simulink model "M4B11"  (R2016b)
settings: Solver=VariableStepAuto  StartTime=0.0  StopTime=25  RelTol=1e-3
InitFcn:
  | initAll
values from neighbouring files (symbols this model uses):
  SgridB = resultsac.baseMVA    [initAll.m]
  wB = 2*pi*fB    (= 314.159265359)    [initAll.m]
undefined symbols (not defined in the file): ACgirdinit, Geninit
libraries: powerlib_meascontrol x4
(part 1 of 2)
settings Model: Creator=LinSiQi  LastModifiedBy=LinSiQi
settings DataIOCC: ReturnWorkspaceOutputs=on
settings SFSimCC: SimUseLocalCustomCode=on
settings RTWCC: RTWUseLocalCustomCode=on

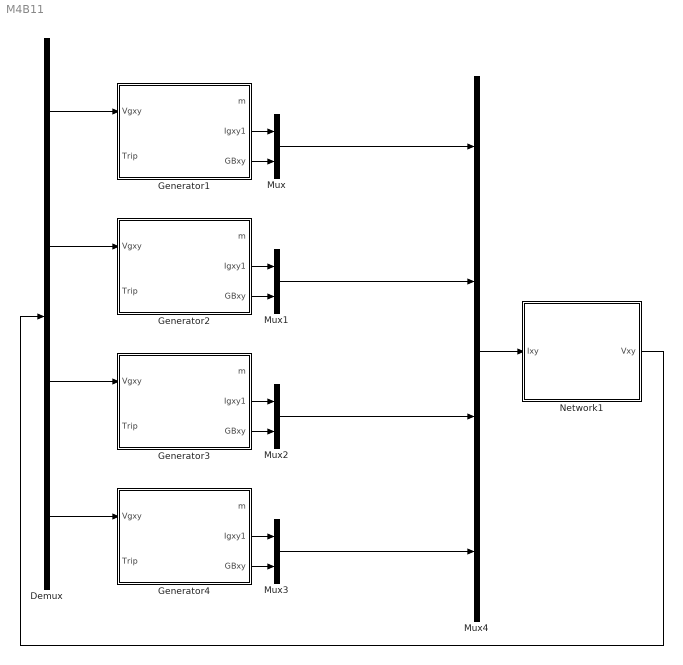
== system M4B11 ==
  Demux : Demux
  Generator1 : Subsystem  mask{wB=wB, SgenB=Geninit.SgenB(1), SgridB=SgridB, Xq=Geninit.Xq(1), Xq1=Geninit.Xq1(1), Xq11=Geninit.Xq11(1), Tq0=Geninit.Tq0(1), Tq10=Geninit.Tq10(1), Eq10=Geninit.Eq1(1), Eq110=Geninit.Eq11(1), Xd=Geninit.Xd(1), Xd1=Geninit.Xd1(1), Xd11=Geninit.Xd11(1), Td0=Geninit.Td0(1), Td10=Geninit.Td10(1), Ed10=Geninit.Ed1(1), Ed110=Geninit.Ed11(1), H=Geninit.Tj(1), D=Geninit.D(1), delta0=Geninit.Delta(1), w0=1, Pm0=Geninit.Pm0(1), Ka=Geninit.Ka(1), Tb=Geninit.Tb(1), Tc=Geninit.Tc(1), Efmin=Geninit.Efmin(1), Efmax=Geninit.Efmax(1), Vref=Geninit.Vref(1), Ef10=Geninit.Vf1(1), S_PSS=Geninit.EnablePSS(1), Kpss=Geninit.kpss(1), Tw_P=Geninit.Tw_P(1), T1_P=Geninit.T1_P(1), T2_P=Geninit.T2_P(1), T3_P=Geninit.T3_P(1), T4_P=Geninit.T4_P(1), Upmax=Geninit.Upmax(1), Upmin=Geninit.Upmin(1), S_Gov=Geninit.Enablegov(1), R=Geninit.R_G(1), Ts_G=Geninit.Ts_G(1), Tc_G=Geninit.Tc_G(1), T3_G=Geninit.T3_G(1), T4_G=Geninit.T4_G(1), T5_G=Geninit.T5_G(1), dPmax=Geninit.dPmax(1), dPmin=Geninit.dPmin(1)}
      mask prompts: S_PSS "Enable PSS"; Tw_P "Tw"; T1_P "T1"; T2_P "T2"; T3_P "T3"; T4_P "T4"; S_Gov "Enable Governor"; Ts_G "Ts"; Tc_G "Tc"; T3_G "T3"; T4_G "T4"; T5_G "T5"
      mask help: This is a six-order synchronous generator with exciter system, governor and PSS.
  Generator2 : Subsystem  mask{wB=wB, SgenB=Geninit.SgenB(2), SgridB=SgridB, Xq=Geninit.Xq(2), Xq1=Geninit.Xq1(2), Xq11=Geninit.Xq11(2), Tq0=Geninit.Tq0(2), Tq10=Geninit.Tq10(2), Eq10=Geninit.Eq1(2), Eq110=Geninit.Eq11(2), Xd=Geninit.Xd(2), Xd1=Geninit.Xd1(2), Xd11=Geninit.Xd11(2), Td0=Geninit.Td0(2), Td10=Geninit.Td10(2), Ed10=Geninit.Ed1(2), Ed110=Geninit.Ed11(2), H=Geninit.Tj(2), D=Geninit.D(2), delta0=Geninit.Delta(2), w0=1, Pm0=Geninit.Pm0(2), Ka=Geninit.Ka(2), Tb=Geninit.Tb(2), Tc=Geninit.Tc(2), Efmin=Geninit.Efmin(2), Efmax=Geninit.Efmax(2), Vref=Geninit.Vref(2), Ef10=Geninit.Vf1(2), S_PSS=Geninit.EnablePSS(2), Kpss=Geninit.kpss(2), Tw_P=Geninit.Tw_P(2), T1_P=Geninit.T1_P(2), T2_P=Geninit.T2_P(2), T3_P=Geninit.T3_P(2), T4_P=Geninit.T4_P(2), Upmax=Geninit.Upmax(2), Upmin=Geninit.Upmin(2), S_Gov=Geninit.Enablegov(2), R=Geninit.R_G(2), Ts_G=Geninit.Ts_G(2), Tc_G=Geninit.Tc_G(2), T3_G=Geninit.T3_G(2), T4_G=Geninit.T4_G(2), T5_G=Geninit.T5_G(2), dPmax=Geninit.dPmax(2), dPmin=Geninit.dPmin(2)}
      mask prompts: S_PSS "Enable PSS"; Tw_P "Tw"; T1_P "T1"; T2_P "T2"; T3_P "T3"; T4_P "T4"; S_Gov "Enable Governor"; Ts_G "Ts"; Tc_G "Tc"; T3_G "T3"; T4_G "T4"; T5_G "T5"
      mask help: This is a six-order synchronous generator with exciter system, governor and PSS.
  Generator3 : Subsystem  mask{wB=wB, SgenB=Geninit.SgenB(3), SgridB=SgridB, Xq=Geninit.Xq(3), Xq1=Geninit.Xq1(3), Xq11=Geninit.Xq11(3), Tq0=Geninit.Tq0(3), Tq10=Geninit.Tq10(3), Eq10=Geninit.Eq1(3), Eq110=Geninit.Eq11(3), Xd=Geninit.Xd(3), Xd1=Geninit.Xd1(3), Xd11=Geninit.Xd11(3), Td0=Geninit.Td0(3), Td10=Geninit.Td10(3), Ed10=Geninit.Ed1(3), Ed110=Geninit.Ed11(3), H=Geninit.Tj(3), D=Geninit.D(3), delta0=Geninit.Delta(3), w0=1, Pm0=Geninit.Pm0(3), Ka=Geninit.Ka(3), Tb=Geninit.Tb(3), Tc=Geninit.Tc(3), Efmin=Geninit.Efmin(3), Efmax=Geninit.Efmax(3), Vref=Geninit.Vref(3), Ef10=Geninit.Vf1(3), S_PSS=Geninit.EnablePSS(3), Kpss=Geninit.kpss(3), Tw_P=Geninit.Tw_P(3), T1_P=Geninit.T1_P(3), T2_P=Geninit.T2_P(3), T3_P=Geninit.T3_P(3), T4_P=Geninit.T4_P(3), Upmax=Geninit.Upmax(3), Upmin=Geninit.Upmin(3), S_Gov=Geninit.Enablegov(3), R=Geninit.R_G(3), Ts_G=Geninit.Ts_G(3), Tc_G=Geninit.Tc_G(3), T3_G=Geninit.T3_G(3), T4_G=Geninit.T4_G(3), T5_G=Geninit.T5_G(3), dPmax=Geninit.dPmax(3), dPmin=Geninit.dPmin(3)}
      mask prompts: S_PSS "Enable PSS"; Tw_P "Tw"; T1_P "T1"; T2_P "T2"; T3_P "T3"; T4_P "T4"; S_Gov "Enable Governor"; Ts_G "Ts"; Tc_G "Tc"; T3_G "T3"; T4_G "T4"; T5_G "T5"
      mask help: This is a six-order synchronous generator with exciter system, governor and PSS.
  Generator4 : Subsystem  mask{wB=wB, SgenB=Geninit.SgenB(4), SgridB=SgridB, Xq=Geninit.Xq(4), Xq1=Geninit.Xq1(4), Xq11=Geninit.Xq11(4), Tq0=Geninit.Tq0(4), Tq10=Geninit.Tq10(4), Eq10=Geninit.Eq1(4), Eq110=Geninit.Eq11(4), Xd=Geninit.Xd(4), Xd1=Geninit.Xd1(4), Xd11=Geninit.Xd11(4), Td0=Geninit.Td0(4), Td10=Geninit.Td10(4), Ed10=Geninit.Ed1(4), Ed110=Geninit.Ed11(4), H=Geninit.Tj(4), D=Geninit.D(4), delta0=Geninit.Delta(4), w0=1, Pm0=Geninit.Pm0(4), Ka=Geninit.Ka(4), Tb=Geninit.Tb(4), Tc=Geninit.Tc(4), Efmin=Geninit.Efmin(4), Efmax=Geninit.Efmax(4), Vref=Geninit.Vref(4), Ef10=Geninit.Vf1(4), S_PSS=Geninit.EnablePSS(4), Kpss=Geninit.kpss(4), Tw_P=Geninit.Tw_P(4), T1_P=Geninit.T1_P(4), T2_P=Geninit.T2_P(4), T3_P=Geninit.T3_P(4), T4_P=Geninit.T4_P(4), Upmax=Geninit.Upmax(4), Upmin=Geninit.Upmin(4), S_Gov=Geninit.Enablegov(4), R=Geninit.R_G(4), Ts_G=Geninit.Ts_G(4), Tc_G=Geninit.Tc_G(4), T3_G=Geninit.T3_G(4), T4_G=Geninit.T4_G(4), T5_G=Geninit.T5_G(4), dPmax=Geninit.dPmax(4), dPmin=Geninit.dPmin(4)}
      mask prompts: S_PSS "Enable PSS"; Tw_P "Tw"; T1_P "T1"; T2_P "T2"; T3_P "T3"; T4_P "T4"; S_Gov "Enable Governor"; Ts_G "Ts"; Tc_G "Tc"; T3_G "T3"; T4_G "T4"; T5_G "T5"
      mask help: This is a six-order synchronous generator with exciter system, governor and PSS.
  Mux{,1..3} (4 alike) : Mux  Inputs=2
  Mux4 : Mux
  Network1 : Subsystem  mask{busdata=ACgirdinit.busdata{1}, linedata=ACgirdinit.linedata{1}, VSS0=ACgirdinit.VSS0{1}, LINE=ACgirdinit.fline{1}, fbus=ACgirdinit.FBUS(1), ng=ACgirdinit.ng{1}, Currentin_idx=ACgirdinit.Currentin_idx{1}}
  wires:
  Mux/1 -> Mux4/1
  Generator2/2(Igxy1) -> Mux1/1
  Generator3/2(Igxy1) -> Mux2/1
  Generator1/2(Igxy1) -> Mux/1
  Generator2/3(GBxy) -> Mux1/2
  Mux1/1 -> Mux4/2
  Mux2/1 -> Mux4/3
  Mux3/1 -> Mux4/4
  Generator4/3(GBxy) -> Mux3/2
  Generator4/2(Igxy1) -> Mux3/1
  Generator1/3(GBxy) -> Mux/2
  Generator3/3(GBxy) -> Mux2/2
  Mux4/1 -> Network1/1(Ixy)
  Demux/1 -> Generator1/1(Vgxy)
  Demux/2 -> Generator2/1(Vgxy)
  Demux/3 -> Generator3/1(Vgxy)
  Demux/4 -> Generator4/1(Vgxy)
  Network1/1(Vxy) -> Demux/1

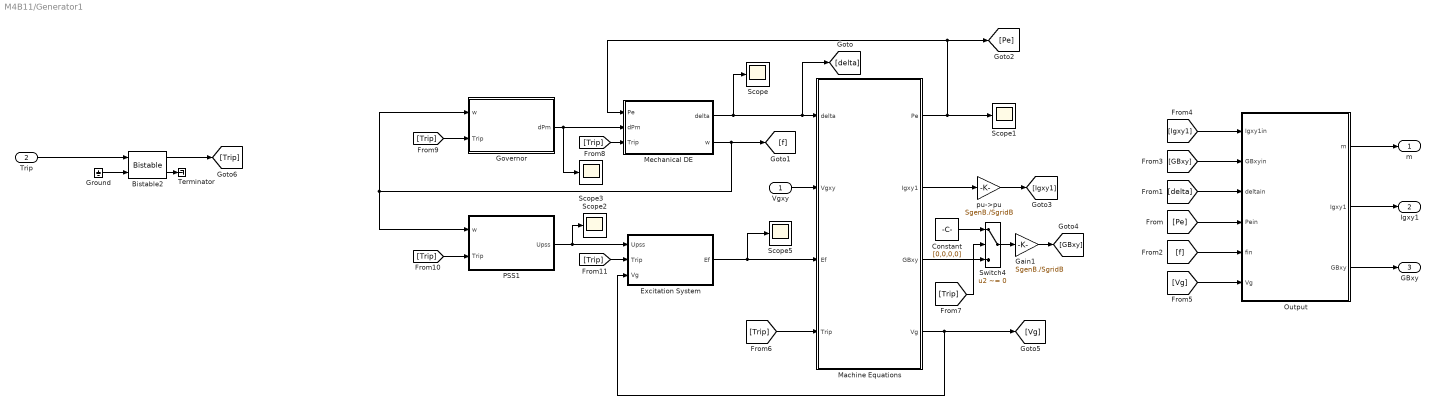
== system M4B11/Generator1 ==
  Vgxy : Inport
  Trip : Inport  Port=2
  Bistable2 : powerlib_meascontrol/Logic/Bistable  Qpriority=Set  ic=0  Ts=0
  Constant : Constant  Value=[0,0,0,0]
  Excitation System : Subsystem
  Gain1 : Gain  Gain=SgenB./SgridB
  Governor : Subsystem
  Ground : Ground
  "Machine Equations " : Subsystem
  Mechanical DE : Subsystem
  Output : Subsystem
  PSS1 : Subsystem
  Scope{,1..3,5} (5 alike) : Scope
  Switch4 : Switch  Criteria=u2 ~= 0  Threshold=0.5  SaturateOnIntegerOverflow=on
  Terminator : Terminator
  pu->pu : Gain  Gain=SgenB./SgridB
  m : Outport
  Igxy1 : Outport  Port=2
  GBxy : Outport  Port=3
  wires:
  Gain1/1 -> [GBxy]
  pu->pu/1 -> [Igxy1]
  [Trip] -> PSS1/2(Trip)
  [Trip] -> Governor/2(Trip)
  [GBxy] -> Output/2(GBxyin)
  [Trip] -> Excitation System/2(Trip)
  Output/1(m) -> m/1
  Mechanical DE/1(delta) -> Scope/1, "Machine Equations "/1(delta), [delta]
  Bistable2/2 -> Terminator/1
  [f] -> Output/5(fin)
  Output/2(Igxy1) -> Igxy1/1
  PSS1/1(Upss) -> Excitation System/1(Upss), Scope2/1
  "Machine Equations "/3(GBxy) -> Switch4/3
  Vgxy/1 -> "Machine Equations "/2(Vgxy)
  Constant/1 -> Switch4/1
  "Machine Equations "/2(Igxy1) -> pu->pu/1
  Governor/1(dPm) -> Mechanical DE/2(dPm), Scope3/1
  [delta] -> Output/3(deltain)
  [Vg] -> Output/6(Vg)
  [Igxy1] -> Output/1(Igxy1in)
  Mechanical DE/2(w) -> Governor/1(w), PSS1/1(w), [f]
  Output/3(GBxy) -> GBxy/1
  Excitation System/1(Ef) -> Scope5/1, "Machine Equations "/3(Ef)
  "Machine Equations "/4(Vg) -> [Vg], Excitation System/3(Vg)
  [Trip] -> "Machine Equations "/4(Trip)
  [Trip] -> Switch4/2
  Bistable2/1 -> [Trip]
  "Machine Equations "/1(Pe) -> Scope1/1, Mechanical DE/1(Pe), [Pe]
  [Pe] -> Output/4(Pein)
  Switch4/1 -> Gain1/1
  Trip/1 -> Bistable2/1
  Ground/1 -> Bistable2/2
  [Trip] -> Mechanical DE/3(Trip)

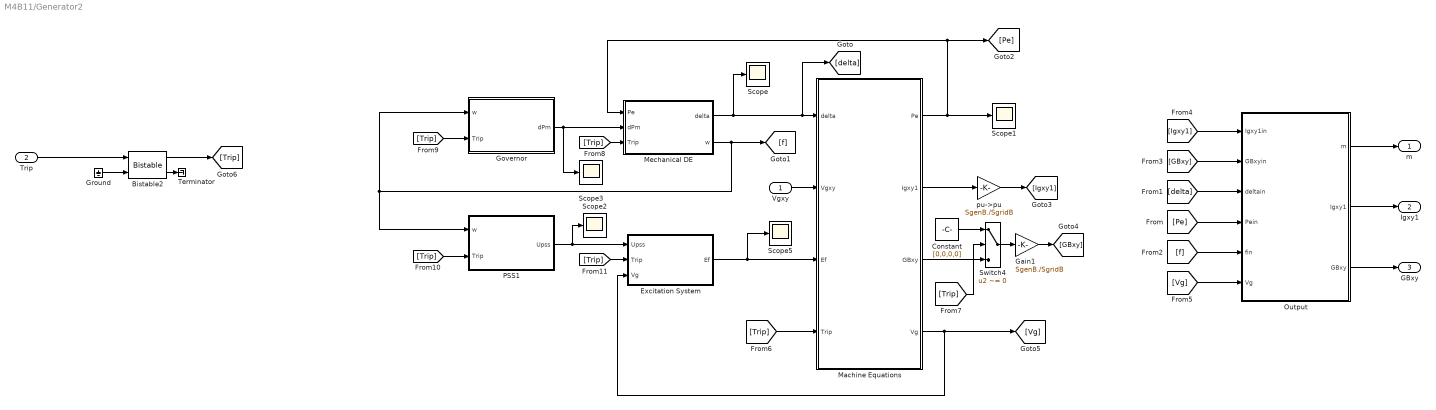
== system M4B11/Generator2 ==
  Vgxy : Inport
  Trip : Inport  Port=2
  Bistable2 : powerlib_meascontrol/Logic/Bistable  Qpriority=Set  ic=0  Ts=0
  Constant : Constant  Value=[0,0,0,0]
  Excitation System : Subsystem
  Gain1 : Gain  Gain=SgenB./SgridB
  Governor : Subsystem
  Ground : Ground
  "Machine Equations " : Subsystem
  Mechanical DE : Subsystem
  Output : Subsystem
  PSS1 : Subsystem
  Scope{,1..3,5} (5 alike) : Scope
  Switch4 : Switch  Criteria=u2 ~= 0  Threshold=0.5  SaturateOnIntegerOverflow=on
  Terminator : Terminator
  pu->pu : Gain  Gain=SgenB./SgridB
  m : Outport
  Igxy1 : Outport  Port=2
  GBxy : Outport  Port=3
  wires:
  Gain1/1 -> [GBxy]
  pu->pu/1 -> [Igxy1]
  [Trip] -> PSS1/2(Trip)
  [Trip] -> Governor/2(Trip)
  [GBxy] -> Output/2(GBxyin)
  [Trip] -> Excitation System/2(Trip)
  Output/1(m) -> m/1
  Mechanical DE/1(delta) -> Scope/1, "Machine Equations "/1(delta), [delta]
  Bistable2/2 -> Terminator/1
  [f] -> Output/5(fin)
  Output/2(Igxy1) -> Igxy1/1
  PSS1/1(Upss) -> Excitation System/1(Upss), Scope2/1
  "Machine Equations "/3(GBxy) -> Switch4/3
  Vgxy/1 -> "Machine Equations "/2(Vgxy)
  Constant/1 -> Switch4/1
  "Machine Equations "/2(Igxy1) -> pu->pu/1
  Governor/1(dPm) -> Mechanical DE/2(dPm), Scope3/1
  [delta] -> Output/3(deltain)
  [Vg] -> Output/6(Vg)
  [Igxy1] -> Output/1(Igxy1in)
  Mechanical DE/2(w) -> Governor/1(w), PSS1/1(w), [f]
  Output/3(GBxy) -> GBxy/1
  Excitation System/1(Ef) -> Scope5/1, "Machine Equations "/3(Ef)
  "Machine Equations "/4(Vg) -> [Vg], Excitation System/3(Vg)
  [Trip] -> "Machine Equations "/4(Trip)
  [Trip] -> Switch4/2
  Bistable2/1 -> [Trip]
  "Machine Equations "/1(Pe) -> Scope1/1, Mechanical DE/1(Pe), [Pe]
  [Pe] -> Output/4(Pein)
  Switch4/1 -> Gain1/1
  Trip/1 -> Bistable2/1
  Ground/1 -> Bistable2/2
  [Trip] -> Mechanical DE/3(Trip)

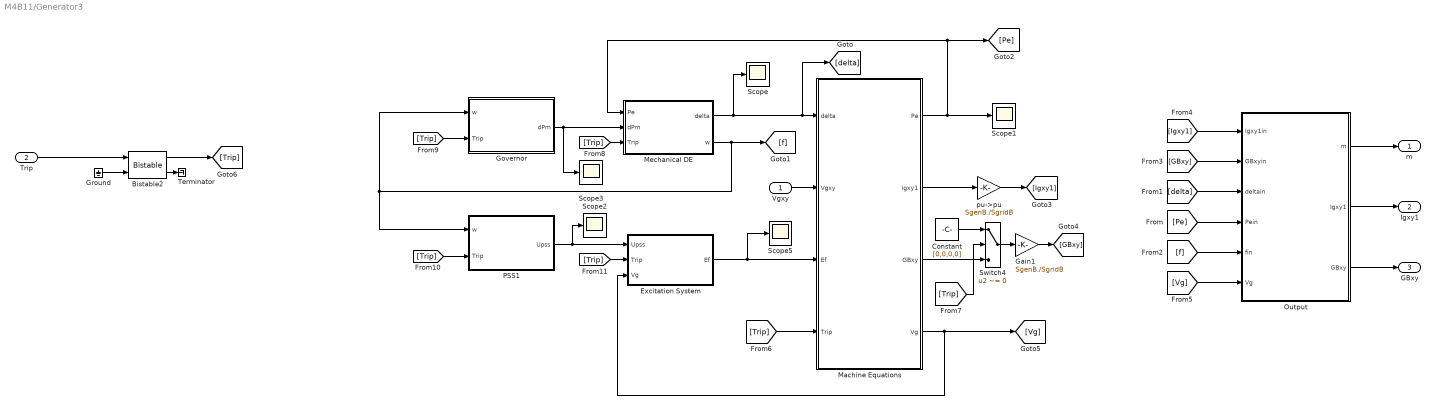
== system M4B11/Generator3 ==
  Vgxy : Inport
  Trip : Inport  Port=2
  Bistable2 : powerlib_meascontrol/Logic/Bistable  Qpriority=Set  ic=0  Ts=0
  Constant : Constant  Value=[0,0,0,0]
  Excitation System : Subsystem
  Gain1 : Gain  Gain=SgenB./SgridB
  Governor : Subsystem
  Ground : Ground
  "Machine Equations " : Subsystem
  Mechanical DE : Subsystem
  Output : Subsystem
  PSS1 : Subsystem
  Scope{,1..3,5} (5 alike) : Scope
  Switch4 : Switch  Criteria=u2 ~= 0  Threshold=0.5  SaturateOnIntegerOverflow=on
  Terminator : Terminator
  pu->pu : Gain  Gain=SgenB./SgridB
  m : Outport
  Igxy1 : Outport  Port=2
  GBxy : Outport  Port=3
  wires:
  Gain1/1 -> [GBxy]
  pu->pu/1 -> [Igxy1]
  [Trip] -> PSS1/2(Trip)
  [Trip] -> Governor/2(Trip)
  [GBxy] -> Output/2(GBxyin)
  [Trip] -> Excitation System/2(Trip)
  Output/1(m) -> m/1
  Mechanical DE/1(delta) -> Scope/1, "Machine Equations "/1(delta), [delta]
  Bistable2/2 -> Terminator/1
  [f] -> Output/5(fin)
  Output/2(Igxy1) -> Igxy1/1
  PSS1/1(Upss) -> Excitation System/1(Upss), Scope2/1
  "Machine Equations "/3(GBxy) -> Switch4/3
  Vgxy/1 -> "Machine Equations "/2(Vgxy)
  Constant/1 -> Switch4/1
  "Machine Equations "/2(Igxy1) -> pu->pu/1
  Governor/1(dPm) -> Mechanical DE/2(dPm), Scope3/1
  [delta] -> Output/3(deltain)
  [Vg] -> Output/6(Vg)
  [Igxy1] -> Output/1(Igxy1in)
  Mechanical DE/2(w) -> Governor/1(w), PSS1/1(w), [f]
  Output/3(GBxy) -> GBxy/1
  Excitation System/1(Ef) -> Scope5/1, "Machine Equations "/3(Ef)
  "Machine Equations "/4(Vg) -> [Vg], Excitation System/3(Vg)
  [Trip] -> "Machine Equations "/4(Trip)
  [Trip] -> Switch4/2
  Bistable2/1 -> [Trip]
  "Machine Equations "/1(Pe) -> Scope1/1, Mechanical DE/1(Pe), [Pe]
  [Pe] -> Output/4(Pein)
  Switch4/1 -> Gain1/1
  Trip/1 -> Bistable2/1
  Ground/1 -> Bistable2/2
  [Trip] -> Mechanical DE/3(Trip)

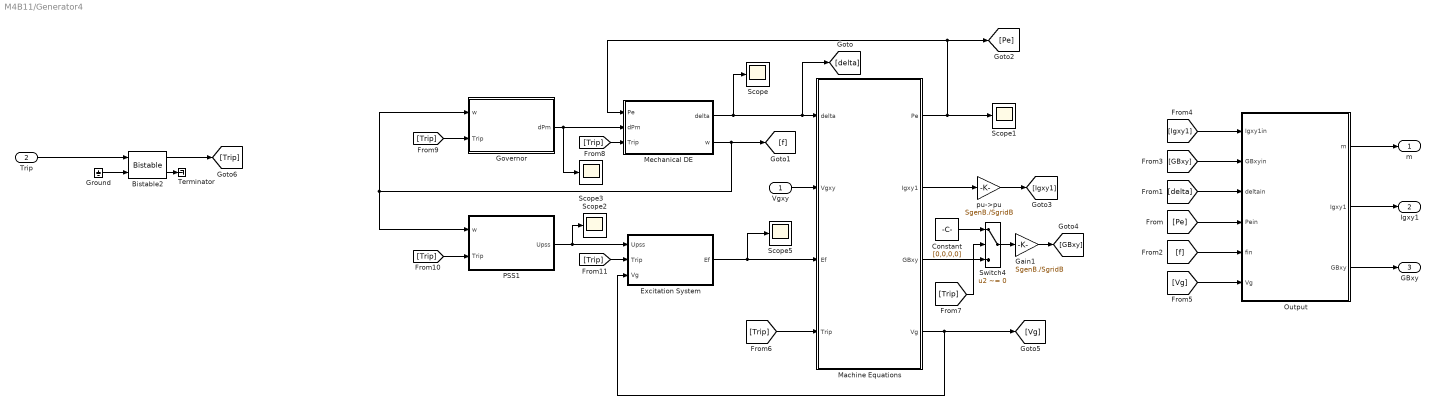
== system M4B11/Generator4 ==
  Vgxy : Inport
  Trip : Inport  Port=2
  Bistable2 : powerlib_meascontrol/Logic/Bistable  Qpriority=Set  ic=0  Ts=0
  Constant : Constant  Value=[0,0,0,0]
  Excitation System : Subsystem
  Gain1 : Gain  Gain=SgenB./SgridB
  Governor : Subsystem
  Ground : Ground
  "Machine Equations " : Subsystem
  Mechanical DE : Subsystem
  Output : Subsystem
  PSS1 : Subsystem
  Scope{,1..3,5} (5 alike) : Scope
  Switch4 : Switch  Criteria=u2 ~= 0  Threshold=0.5  SaturateOnIntegerOverflow=on
  Terminator : Terminator
  pu->pu : Gain  Gain=SgenB./SgridB
  m : Outport
  Igxy1 : Outport  Port=2
  GBxy : Outport  Port=3
  wires:
  Gain1/1 -> [GBxy]
  pu->pu/1 -> [Igxy1]
  [Trip] -> PSS1/2(Trip)
  [Trip] -> Governor/2(Trip)
  [GBxy] -> Output/2(GBxyin)
  [Trip] -> Excitation System/2(Trip)
  Output/1(m) -> m/1
  Mechanical DE/1(delta) -> Scope/1, "Machine Equations "/1(delta), [delta]
  Bistable2/2 -> Terminator/1
  [f] -> Output/5(fin)
  Output/2(Igxy1) -> Igxy1/1
  PSS1/1(Upss) -> Excitation System/1(Upss), Scope2/1
  "Machine Equations "/3(GBxy) -> Switch4/3
  Vgxy/1 -> "Machine Equations "/2(Vgxy)
  Constant/1 -> Switch4/1
  "Machine Equations "/2(Igxy1) -> pu->pu/1
  Governor/1(dPm) -> Mechanical DE/2(dPm), Scope3/1
  [delta] -> Output/3(deltain)
  [Vg] -> Output/6(Vg)
  [Igxy1] -> Output/1(Igxy1in)
  Mechanical DE/2(w) -> Governor/1(w), PSS1/1(w), [f]
  Output/3(GBxy) -> GBxy/1
  Excitation System/1(Ef) -> Scope5/1, "Machine Equations "/3(Ef)
  "Machine Equations "/4(Vg) -> [Vg], Excitation System/3(Vg)
  [Trip] -> "Machine Equations "/4(Trip)
  [Trip] -> Switch4/2
  Bistable2/1 -> [Trip]
  "Machine Equations "/1(Pe) -> Scope1/1, Mechanical DE/1(Pe), [Pe]
  [Pe] -> Output/4(Pein)
  Switch4/1 -> Gain1/1
  Trip/1 -> Bistable2/1
  Ground/1 -> Bistable2/2
  [Trip] -> Mechanical DE/3(Trip)

== system M4B11/Network1 ==
  Ixy : Inport
  Clock : Clock
  Mux : Mux  Inputs=2
  S-Function : S-Function  FunctionName=TS_net_1_new  Parameters=busdata,linedata,VSS0,LINE,fbus,ng,Currentin_idx  SFunctionDeploymentMode=off  EnableBusSupport=off
  Vxy : Outport
  wires:
  Clock/1 -> Mux/1
  Ixy/1 -> Mux/2
  Mux/1 -> S-Function/1
  S-Function/1 -> Vxy/1

== system M4B11/Generator1/Excitation System ==
  note: Ef
  Upss : Inport
  Trip : Inport  Port=2
  Vg : Inport  Port=3
  Constant : Constant  Value=0
  KA : Gain  Gain=Ka  SaturateOnIntegerOverflow=on  OutDataTypeStr=Inherit: Same as input  ParamDataTypeStr=Inherit: Same as input
  Saturation : Saturate  UpperLimit=Efmax  LowerLimit=Efmin
  Scope : Scope  NumInputPorts=2
  Sum4 : Sum  Inputs=+-+  SaturateOnIntegerOverflow=on
  Switch : Switch  Criteria=u2 ~= 0  Threshold=0.5  SaturateOnIntegerOverflow=on
  Vref : Constant  Value=Vref
  Ef : Outport
  wires:
  Trip/1 -> Switch/2
  Constant/1 -> Switch/1
  Switch/1 -> Ef/1
  Saturation/1 -> Switch/3
  Sum4/1 -> KA/1
  KA/1 -> Saturation/1
  Vg/1 -> Sum4/2, Scope/2
  Upss/1 -> Sum4/3
  Vref/1 -> Scope/1, Sum4/1

== system M4B11/Generator1/Governor ==
  w : Inport
  Trip : Inport  Port=2
  CT : Constant  Value=0
  Constant : Constant  Value=0
  Gain1 : Gain  Gain=1/R  SaturateOnIntegerOverflow=on  OutDataTypeStr=Inherit: Same as input  ParamDataTypeStr=Inherit: Same as input
  Saturation : Saturate  UpperLimit=dPmax  LowerLimit=dPmin
  Sum3 : Sum  Inputs=|+-  SaturateOnIntegerOverflow=on
  Switch : Switch  Threshold=0.5  SaturateOnIntegerOverflow=on
  Switch1 : Switch  Criteria=u2 ~= 0  Threshold=0.5  SaturateOnIntegerOverflow=on
  Transfer Fcn1 : TransferFcn  Denominator=[Ts_G 1]
  Transfer Fcn2 : TransferFcn  Numerator=[T3_G 1]  Denominator=[Tc_G 1]
  Transfer Fcn3 : TransferFcn  Numerator=[T4_G 1]  Denominator=[T5_G 1]
  w1 : Constant  Value=S_Gov
  wref : Constant
  dPm : Outport
  wires:
  Constant/1 -> Switch1/1
  Switch/1 -> Switch1/3
  Trip/1 -> Switch1/2
  Switch1/1 -> dPm/1
  CT/1 -> Switch/3
  w1/1 -> Switch/2
  wref/1 -> Sum3/1
  w/1 -> Sum3/2
  Saturation/1 -> Switch/1
  Sum3/1 -> Gain1/1
  Gain1/1 -> Transfer Fcn1/1
  Transfer Fcn1/1 -> Transfer Fcn2/1
  Transfer Fcn2/1 -> Transfer Fcn3/1
  Transfer Fcn3/1 -> Saturation/1

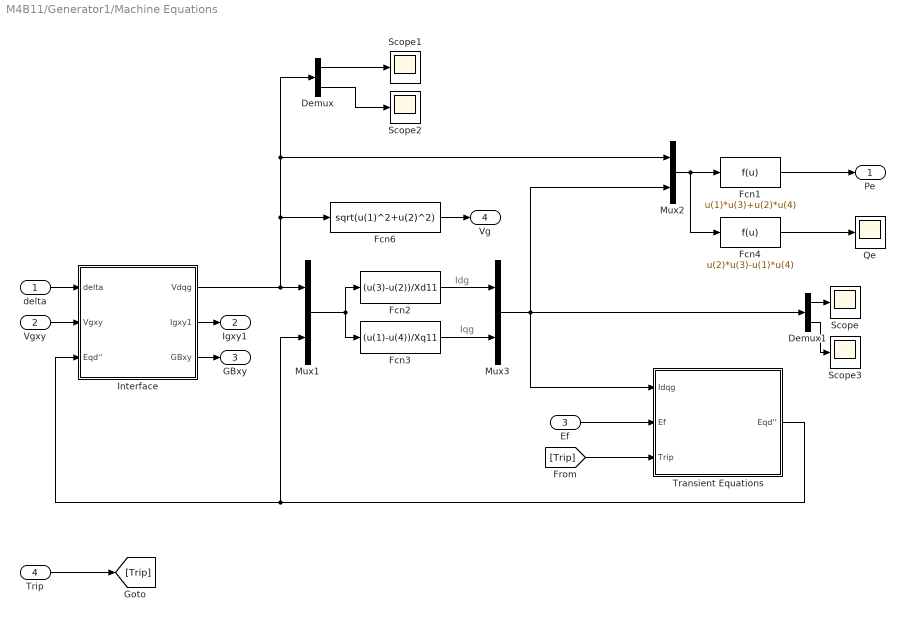
== system M4B11/Generator1/Machine Equations  ==
  note: Idg
  note: Iqg
  delta : Inport
  Vgxy : Inport  Port=2
  Ef : Inport  Port=3
  Trip : Inport  Port=4
  Demux : Demux  Outputs=2
  Demux1 : Demux  Outputs=2
  Fcn1 : Fcn  Expr=u(1)*u(3)+u(2)*u(4)
  Fcn2 : Fcn  Expr=(u(3)-u(2))/Xd11
  Fcn3 : Fcn  Expr=(u(1)-u(4))/Xq11
  Fcn4 : Fcn  Expr=u(2)*u(3)-u(1)*u(4)
  Fcn6 : Fcn  Expr=sqrt(u(1)^2+u(2)^2)
  Interface : Subsystem
  Mux1 : Mux  Inputs=2
  Mux2 : Mux  Inputs=2
  Mux3 : Mux  Inputs=2
  Qe : Scope
  Scope{,1..3} (4 alike) : Scope
  Transient Equations : Subsystem
  Pe : Outport
  Igxy1 : Outport  Port=2
  GBxy : Outport  Port=3
  Vg : Outport  Port=4
  wires:
  Fcn3/1 -> Mux3/2
  Fcn2/1 -> Mux3/1
  Mux3/1 -> Demux1/1, Mux2/2, Transient Equations/1(Idqg)
  Interface/1(Vdqg) -> Demux/1, Mux2/1, Fcn6/1, Mux1/1
  Mux1/1 -> Fcn2/1, Fcn3/1
  Mux2/1 -> Fcn1/1, Fcn4/1
  Ef/1 -> Transient Equations/2(Ef)
  Fcn1/1 -> Pe/1
  Fcn6/1 -> Vg/1
  Fcn4/1 -> Qe/1
  delta/1 -> Interface/1(delta)
  Vgxy/1 -> Interface/2(Vgxy)
  Interface/2(Igxy1) -> Igxy1/1
  Interface/3(GBxy) -> GBxy/1
  Transient Equations/1(Eqd'') -> Mux1/2, Interface/3(Eqd'')
  Demux/1 -> Scope1/1
  Demux1/1 -> Scope/1
  Demux/2 -> Scope2/1
  Demux1/2 -> Scope3/1
  Trip/1 -> [Trip]
  [Trip] -> Transient Equations/3(Trip)

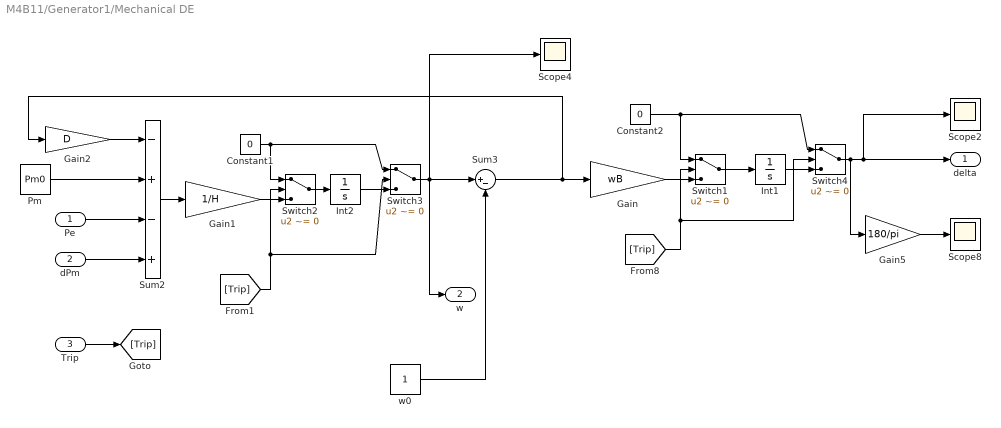
== system M4B11/Generator1/Mechanical DE ==
  Pe : Inport
  dPm : Inport  Port=2
  Trip : Inport  Port=3
  Constant1 : Constant  Value=0
  Constant2 : Constant  Value=0
  Gain : Gain  Gain=wB  SaturateOnIntegerOverflow=on  OutDataTypeStr=Inherit: Same as input  ParamDataTypeStr=Inherit: Same as input
  Gain1 : Gain  Gain=1/H  SaturateOnIntegerOverflow=on  OutDataTypeStr=Inherit: Same as input  ParamDataTypeStr=Inherit: Same as input
  Gain2 : Gain  Gain=D  SaturateOnIntegerOverflow=on  OutDataTypeStr=Inherit: Same as input  ParamDataTypeStr=Inherit: Same as input
  Gain5 : Gain  Gain=180/pi  SaturateOnIntegerOverflow=on  OutDataTypeStr=Inherit: Same as input  ParamDataTypeStr=Inherit: Same as input
  Int1 : Integrator  InitialCondition=delta0
  Int2 : Integrator  InitialCondition=w0
  Pm : Constant  Value=Pm0
  Scope2 : Scope
  Scope4 : Scope
  Scope8 : Scope
  Sum2 : Sum  Inputs=-+-+  SaturateOnIntegerOverflow=on
  Sum3 : Sum  Inputs=|+-  SaturateOnIntegerOverflow=on
  Switch{1..4} (4 alike) : Switch  Criteria=u2 ~= 0  Threshold=0.5  SaturateOnIntegerOverflow=on
  w0 : Constant
  delta : Outport
  w : Outport  Port=2
  wires:
  [Trip] -> Switch3/2, Switch2/2
  Constant1/1 -> Switch3/1, Switch2/1
  Switch3/1 -> Scope4/1, Sum3/1, w/1
  Int2/1 -> Switch3/3
  Switch2/1 -> Int2/1
  Gain1/1 -> Switch2/3
  Trip/1 -> [Trip]
  [Trip] -> Switch1/2, Switch4/2
  Constant2/1 -> Switch4/1, Switch1/1
  Switch4/1 -> delta/1, Scope2/1, Gain5/1
  Int1/1 -> Switch4/3
  Switch1/1 -> Int1/1
  Gain/1 -> Switch1/3
  Gain5/1 -> Scope8/1
  w0/1 -> Sum3/2
  Sum3/1 -> Gain2/1, Gain/1
  Pm/1 -> Sum2/2
  Gain2/1 -> Sum2/1
  Sum2/1 -> Gain1/1
  Pe/1 -> Sum2/3
  dPm/1 -> Sum2/4

== system M4B11/Generator1/Output ==
  Igxy1in : Inport
  GBxyin : Inport  Port=2
  deltain : Inport  Port=3
  Pein : Inport  Port=4
  fin : Inport  Port=5
  Vg : Inport  Port=6
  Bus Creator : BusCreator  Inputs=6
  m : Outport
  Igxy1 : Outport  Port=2
  GBxy : Outport  Port=3
  wires:
  Bus Creator/1 -> m/1
  Igxy1in/1 -> Igxy1/1, Bus Creator/1  "Igxy1"
  GBxyin/1 -> GBxy/1, Bus Creator/2  "GBxy"
  deltain/1 -> Bus Creator/3  "delta"
  Pein/1 -> Bus Creator/4  "Pe"
  fin/1 -> Bus Creator/5  "f"
  Vg/1 -> Bus Creator/6  "Vg"

== system M4B11/Generator1/PSS1 ==
  w : Inport
  Trip : Inport  Port=2
  CT : Constant  Value=0
  Constant : Constant  Value=0
  Gain : Gain  Gain=Kpss  SaturateOnIntegerOverflow=on  OutDataTypeStr=Inherit: Same as input  ParamDataTypeStr=Inherit: Same as input
  Saturation : Saturate  UpperLimit=Upmax  LowerLimit=Upmin
  Sum3 : Sum  Inputs=|+-  SaturateOnIntegerOverflow=on
  Switch : Switch  Threshold=0.5  SaturateOnIntegerOverflow=on
  Switch1 : Switch  Threshold=0.5  SaturateOnIntegerOverflow=on
  Transfer Fcn : TransferFcn  Numerator=[Tw_P 0]  Denominator=[Tw_P 1]
  Transfer Fcn1 : TransferFcn  Numerator=[T1_P 1]  Denominator=[T2_P 1]
  Transfer Fcn2 : TransferFcn  Numerator=[T3_P 1]  Denominator=[T4_P 1]
  w0 : Constant
  w1 : Constant  Value=S_PSS
  Upss : Outport
  wires:
  Constant/1 -> Switch1/1
  Trip/1 -> Switch1/2
  Switch1/1 -> Upss/1
  Switch/1 -> Switch1/3
  Transfer Fcn/1 -> Transfer Fcn1/1
  Gain/1 -> Transfer Fcn/1
  w1/1 -> Switch/2
  CT/1 -> Switch/3
  Saturation/1 -> Switch/1
  Sum3/1 -> Gain/1
  Transfer Fcn2/1 -> Saturation/1
  Transfer Fcn1/1 -> Transfer Fcn2/1
  w/1 -> Sum3/1
  w0/1 -> Sum3/2

== system M4B11/Generator2/Excitation System ==
  note: Ef
  Upss : Inport
  Trip : Inport  Port=2
  Vg : Inport  Port=3
  Constant : Constant  Value=0
  KA : Gain  Gain=Ka  SaturateOnIntegerOverflow=on  OutDataTypeStr=Inherit: Same as input  ParamDataTypeStr=Inherit: Same as input
  Saturation : Saturate  UpperLimit=Efmax  LowerLimit=Efmin
  Scope : Scope  NumInputPorts=2
  Sum4 : Sum  Inputs=+-+  SaturateOnIntegerOverflow=on
  Switch : Switch  Criteria=u2 ~= 0  Threshold=0.5  SaturateOnIntegerOverflow=on
  Vref : Constant  Value=Vref
  Ef : Outport
  wires:
  Trip/1 -> Switch/2
  Constant/1 -> Switch/1
  Switch/1 -> Ef/1
  Saturation/1 -> Switch/3
  Sum4/1 -> KA/1
  KA/1 -> Saturation/1
  Vg/1 -> Sum4/2, Scope/2
  Upss/1 -> Sum4/3
  Vref/1 -> Scope/1, Sum4/1

== system M4B11/Generator2/Governor ==
  w : Inport
  Trip : Inport  Port=2
  CT : Constant  Value=0
  Constant : Constant  Value=0
  Gain1 : Gain  Gain=1/R  SaturateOnIntegerOverflow=on  OutDataTypeStr=Inherit: Same as input  ParamDataTypeStr=Inherit: Same as input
  Saturation : Saturate  UpperLimit=dPmax  LowerLimit=dPmin
  Sum3 : Sum  Inputs=|+-  SaturateOnIntegerOverflow=on
  Switch : Switch  Threshold=0.5  SaturateOnIntegerOverflow=on
  Switch1 : Switch  Criteria=u2 ~= 0  Threshold=0.5  SaturateOnIntegerOverflow=on
  Transfer Fcn1 : TransferFcn  Denominator=[Ts_G 1]
  Transfer Fcn2 : TransferFcn  Numerator=[T3_G 1]  Denominator=[Tc_G 1]
  Transfer Fcn3 : TransferFcn  Numerator=[T4_G 1]  Denominator=[T5_G 1]
  w1 : Constant  Value=S_Gov
  wref : Constant
  dPm : Outport
  wires:
  Constant/1 -> Switch1/1
  Switch/1 -> Switch1/3
  Trip/1 -> Switch1/2
  Switch1/1 -> dPm/1
  CT/1 -> Switch/3
  w1/1 -> Switch/2
  wref/1 -> Sum3/1
  w/1 -> Sum3/2
  Saturation/1 -> Switch/1
  Sum3/1 -> Gain1/1
  Gain1/1 -> Transfer Fcn1/1
  Transfer Fcn1/1 -> Transfer Fcn2/1
  Transfer Fcn2/1 -> Transfer Fcn3/1
  Transfer Fcn3/1 -> Saturation/1

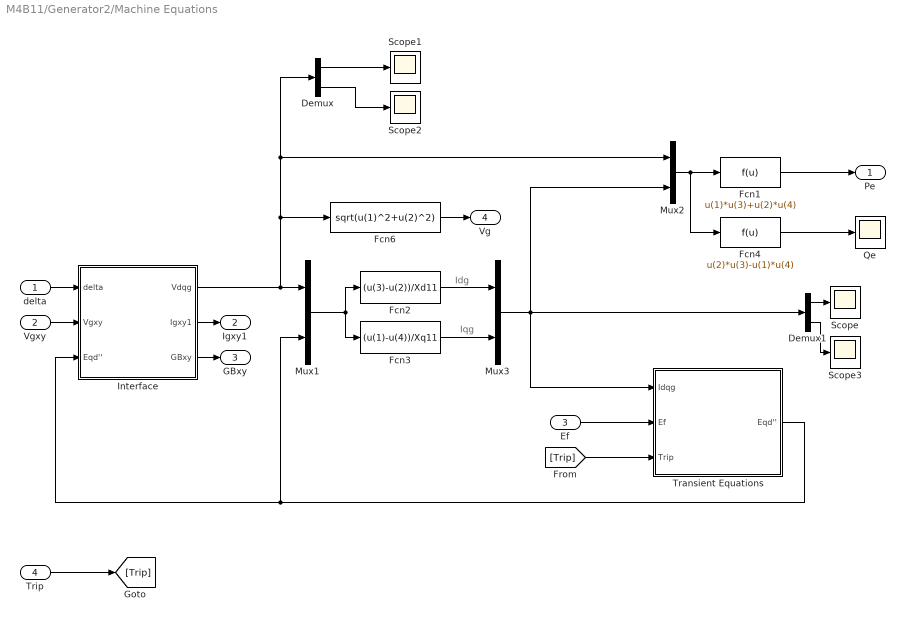
== system M4B11/Generator2/Machine Equations  ==
  note: Idg
  note: Iqg
  delta : Inport
  Vgxy : Inport  Port=2
  Ef : Inport  Port=3
  Trip : Inport  Port=4
  Demux : Demux  Outputs=2
  Demux1 : Demux  Outputs=2
  Fcn1 : Fcn  Expr=u(1)*u(3)+u(2)*u(4)
  Fcn2 : Fcn  Expr=(u(3)-u(2))/Xd11
  Fcn3 : Fcn  Expr=(u(1)-u(4))/Xq11
  Fcn4 : Fcn  Expr=u(2)*u(3)-u(1)*u(4)
  Fcn6 : Fcn  Expr=sqrt(u(1)^2+u(2)^2)
  Interface : Subsystem
  Mux1 : Mux  Inputs=2
  Mux2 : Mux  Inputs=2
  Mux3 : Mux  Inputs=2
  Qe : Scope
  Scope{,1..3} (4 alike) : Scope
  Transient Equations : Subsystem
  Pe : Outport
  Igxy1 : Outport  Port=2
  GBxy : Outport  Port=3
  Vg : Outport  Port=4
  wires:
  Fcn3/1 -> Mux3/2
  Fcn2/1 -> Mux3/1
  Mux3/1 -> Demux1/1, Mux2/2, Transient Equations/1(Idqg)
  Interface/1(Vdqg) -> Demux/1, Mux2/1, Fcn6/1, Mux1/1
  Mux1/1 -> Fcn2/1, Fcn3/1
  Mux2/1 -> Fcn1/1, Fcn4/1
  Ef/1 -> Transient Equations/2(Ef)
  Fcn1/1 -> Pe/1
  Fcn6/1 -> Vg/1
  Fcn4/1 -> Qe/1
  delta/1 -> Interface/1(delta)
  Vgxy/1 -> Interface/2(Vgxy)
  Interface/2(Igxy1) -> Igxy1/1
  Interface/3(GBxy) -> GBxy/1
  Transient Equations/1(Eqd'') -> Mux1/2, Interface/3(Eqd'')
  Demux/1 -> Scope1/1
  Demux1/1 -> Scope/1
  Demux/2 -> Scope2/1
  Demux1/2 -> Scope3/1
  Trip/1 -> [Trip]
  [Trip] -> Transient Equations/3(Trip)

== system M4B11/Generator2/Mechanical DE ==
  Pe : Inport
  dPm : Inport  Port=2
  Trip : Inport  Port=3
  Constant1 : Constant  Value=0
  Constant2 : Constant  Value=0
  Gain : Gain  Gain=wB  SaturateOnIntegerOverflow=on  OutDataTypeStr=Inherit: Same as input  ParamDataTypeStr=Inherit: Same as input
  Gain1 : Gain  Gain=1/H  SaturateOnIntegerOverflow=on  OutDataTypeStr=Inherit: Same as input  ParamDataTypeStr=Inherit: Same as input
  Gain2 : Gain  Gain=D  SaturateOnIntegerOverflow=on  OutDataTypeStr=Inherit: Same as input  ParamDataTypeStr=Inherit: Same as input
  Gain5 : Gain  Gain=180/pi  SaturateOnIntegerOverflow=on  OutDataTypeStr=Inherit: Same as input  ParamDataTypeStr=Inherit: Same as input
  Int1 : Integrator  InitialCondition=delta0
  Int2 : Integrator  InitialCondition=w0
  Pm : Constant  Value=Pm0
  Scope2 : Scope
  Scope4 : Scope
  Scope8 : Scope
  Sum2 : Sum  Inputs=-+-+  SaturateOnIntegerOverflow=on
  Sum3 : Sum  Inputs=|+-  SaturateOnIntegerOverflow=on
  Switch{1..4} (4 alike) : Switch  Criteria=u2 ~= 0  Threshold=0.5  SaturateOnIntegerOverflow=on
  w0 : Constant
  delta : Outport
  w : Outport  Port=2
  wires:
  [Trip] -> Switch3/2, Switch2/2
  Constant1/1 -> Switch3/1, Switch2/1
  Switch3/1 -> Scope4/1, Sum3/1, w/1
  Int2/1 -> Switch3/3
  Switch2/1 -> Int2/1
  Gain1/1 -> Switch2/3
  Trip/1 -> [Trip]
  [Trip] -> Switch1/2, Switch4/2
  Constant2/1 -> Switch4/1, Switch1/1
  Switch4/1 -> delta/1, Scope2/1, Gain5/1
  Int1/1 -> Switch4/3
  Switch1/1 -> Int1/1
  Gain/1 -> Switch1/3
  Gain5/1 -> Scope8/1
  w0/1 -> Sum3/2
  Sum3/1 -> Gain2/1, Gain/1
  Pm/1 -> Sum2/2
  Gain2/1 -> Sum2/1
  Sum2/1 -> Gain1/1
  Pe/1 -> Sum2/3
  dPm/1 -> Sum2/4

== system M4B11/Generator2/Output ==
  Igxy1in : Inport
  GBxyin : Inport  Port=2
  deltain : Inport  Port=3
  Pein : Inport  Port=4
  fin : Inport  Port=5
  Vg : Inport  Port=6
  Bus Creator : BusCreator  Inputs=6
  m : Outport
  Igxy1 : Outport  Port=2
  GBxy : Outport  Port=3
  wires:
  Bus Creator/1 -> m/1
  Igxy1in/1 -> Igxy1/1, Bus Creator/1  "Igxy1"
  GBxyin/1 -> GBxy/1, Bus Creator/2  "GBxy"
  deltain/1 -> Bus Creator/3  "delta"
  Pein/1 -> Bus Creator/4  "Pe"
  fin/1 -> Bus Creator/5  "f"
  Vg/1 -> Bus Creator/6  "Vg"

== system M4B11/Generator2/PSS1 ==
  w : Inport
  Trip : Inport  Port=2
  CT : Constant  Value=0
  Constant : Constant  Value=0
  Gain : Gain  Gain=Kpss  SaturateOnIntegerOverflow=on  OutDataTypeStr=Inherit: Same as input  ParamDataTypeStr=Inherit: Same as input
  Saturation : Saturate  UpperLimit=Upmax  LowerLimit=Upmin
  Sum3 : Sum  Inputs=|+-  SaturateOnIntegerOverflow=on
  Switch : Switch  Threshold=0.5  SaturateOnIntegerOverflow=on
  Switch1 : Switch  Threshold=0.5  SaturateOnIntegerOverflow=on
  Transfer Fcn : TransferFcn  Numerator=[Tw_P 0]  Denominator=[Tw_P 1]
  Transfer Fcn1 : TransferFcn  Numerator=[T1_P 1]  Denominator=[T2_P 1]
  Transfer Fcn2 : TransferFcn  Numerator=[T3_P 1]  Denominator=[T4_P 1]
  w0 : Constant
  w1 : Constant  Value=S_PSS
  Upss : Outport
  wires:
  Constant/1 -> Switch1/1
  Trip/1 -> Switch1/2
  Switch1/1 -> Upss/1
  Switch/1 -> Switch1/3
  Transfer Fcn/1 -> Transfer Fcn1/1
  Gain/1 -> Transfer Fcn/1
  w1/1 -> Switch/2
  CT/1 -> Switch/3
  Saturation/1 -> Switch/1
  Sum3/1 -> Gain/1
  Transfer Fcn2/1 -> Saturation/1
  Transfer Fcn1/1 -> Transfer Fcn2/1
  w/1 -> Sum3/1
  w0/1 -> Sum3/2

== system M4B11/Generator3/Excitation System ==
  note: Ef
  Upss : Inport
  Trip : Inport  Port=2
  Vg : Inport  Port=3
  Constant : Constant  Value=0
  KA : Gain  Gain=Ka  SaturateOnIntegerOverflow=on  OutDataTypeStr=Inherit: Same as input  ParamDataTypeStr=Inherit: Same as input
  Saturation : Saturate  UpperLimit=Efmax  LowerLimit=Efmin
  Scope : Scope  NumInputPorts=2
  Sum4 : Sum  Inputs=+-+  SaturateOnIntegerOverflow=on
  Switch : Switch  Criteria=u2 ~= 0  Threshold=0.5  SaturateOnIntegerOverflow=on
  Vref : Constant  Value=Vref
  Ef : Outport
  wires:
  Trip/1 -> Switch/2
  Constant/1 -> Switch/1
  Switch/1 -> Ef/1
  Saturation/1 -> Switch/3
  Sum4/1 -> KA/1
  KA/1 -> Saturation/1
  Vg/1 -> Sum4/2, Scope/2
  Upss/1 -> Sum4/3
  Vref/1 -> Scope/1, Sum4/1

== system M4B11/Generator3/Governor ==
  w : Inport
  Trip : Inport  Port=2
  CT : Constant  Value=0
  Constant : Constant  Value=0
  Gain1 : Gain  Gain=1/R  SaturateOnIntegerOverflow=on  OutDataTypeStr=Inherit: Same as input  ParamDataTypeStr=Inherit: Same as input
  Saturation : Saturate  UpperLimit=dPmax  LowerLimit=dPmin
  Sum3 : Sum  Inputs=|+-  SaturateOnIntegerOverflow=on
  Switch : Switch  Threshold=0.5  SaturateOnIntegerOverflow=on
  Switch1 : Switch  Criteria=u2 ~= 0  Threshold=0.5  SaturateOnIntegerOverflow=on
  Transfer Fcn1 : TransferFcn  Denominator=[Ts_G 1]
  Transfer Fcn2 : TransferFcn  Numerator=[T3_G 1]  Denominator=[Tc_G 1]
  Transfer Fcn3 : TransferFcn  Numerator=[T4_G 1]  Denominator=[T5_G 1]
  w1 : Constant  Value=S_Gov
  wref : Constant
  dPm : Outport
  wires:
  Constant/1 -> Switch1/1
  Switch/1 -> Switch1/3
  Trip/1 -> Switch1/2
  Switch1/1 -> dPm/1
  CT/1 -> Switch/3
  w1/1 -> Switch/2
  wref/1 -> Sum3/1
  w/1 -> Sum3/2
  Saturation/1 -> Switch/1
  Sum3/1 -> Gain1/1
  Gain1/1 -> Transfer Fcn1/1
  Transfer Fcn1/1 -> Transfer Fcn2/1
  Transfer Fcn2/1 -> Transfer Fcn3/1
  Transfer Fcn3/1 -> Saturation/1

== system M4B11/Generator3/Machine Equations  ==
  note: Idg
  note: Iqg
  delta : Inport
  Vgxy : Inport  Port=2
  Ef : Inport  Port=3
  Trip : Inport  Port=4
  Demux : Demux  Outputs=2
  Demux1 : Demux  Outputs=2
  Fcn1 : Fcn  Expr=u(1)*u(3)+u(2)*u(4)
  Fcn2 : Fcn  Expr=(u(3)-u(2))/Xd11
  Fcn3 : Fcn  Expr=(u(1)-u(4))/Xq11
  Fcn4 : Fcn  Expr=u(2)*u(3)-u(1)*u(4)
  Fcn6 : Fcn  Expr=sqrt(u(1)^2+u(2)^2)
  Interface : Subsystem
  Mux1 : Mux  Inputs=2
  Mux2 : Mux  Inputs=2
  Mux3 : Mux  Inputs=2
  Qe : Scope
  Scope{,1..3} (4 alike) : Scope
  Transient Equations : Subsystem
  Pe : Outport
  Igxy1 : Outport  Port=2
  GBxy : Outport  Port=3
  Vg : Outport  Port=4
  wires:
  Fcn3/1 -> Mux3/2
  Fcn2/1 -> Mux3/1
  Mux3/1 -> Demux1/1, Mux2/2, Transient Equations/1(Idqg)
  Interface/1(Vdqg) -> Demux/1, Mux2/1, Fcn6/1, Mux1/1
  Mux1/1 -> Fcn2/1, Fcn3/1
  Mux2/1 -> Fcn1/1, Fcn4/1
  Ef/1 -> Transient Equations/2(Ef)
  Fcn1/1 -> Pe/1
  Fcn6/1 -> Vg/1
  Fcn4/1 -> Qe/1
  delta/1 -> Interface/1(delta)
  Vgxy/1 -> Interface/2(Vgxy)
  Interface/2(Igxy1) -> Igxy1/1
  Interface/3(GBxy) -> GBxy/1
  Transient Equations/1(Eqd'') -> Mux1/2, Interface/3(Eqd'')
  Demux/1 -> Scope1/1
  Demux1/1 -> Scope/1
  Demux/2 -> Scope2/1
  Demux1/2 -> Scope3/1
  Trip/1 -> [Trip]
  [Trip] -> Transient Equations/3(Trip)

== system M4B11/Generator3/Mechanical DE ==
  Pe : Inport
  dPm : Inport  Port=2
  Trip : Inport  Port=3
  Constant1 : Constant  Value=0
  Constant2 : Constant  Value=0
  Gain : Gain  Gain=wB  SaturateOnIntegerOverflow=on  OutDataTypeStr=Inherit: Same as input  ParamDataTypeStr=Inherit: Same as input
  Gain1 : Gain  Gain=1/H  SaturateOnIntegerOverflow=on  OutDataTypeStr=Inherit: Same as input  ParamDataTypeStr=Inherit: Same as input
  Gain2 : Gain  Gain=D  SaturateOnIntegerOverflow=on  OutDataTypeStr=Inherit: Same as input  ParamDataTypeStr=Inherit: Same as input
  Gain5 : Gain  Gain=180/pi  SaturateOnIntegerOverflow=on  OutDataTypeStr=Inherit: Same as input  ParamDataTypeStr=Inherit: Same as input
  Int1 : Integrator  InitialCondition=delta0
  Int2 : Integrator  InitialCondition=w0
  Pm : Constant  Value=Pm0
  Scope2 : Scope
  Scope4 : Scope
  Scope8 : Scope
  Sum2 : Sum  Inputs=-+-+  SaturateOnIntegerOverflow=on
  Sum3 : Sum  Inputs=|+-  SaturateOnIntegerOverflow=on
  Switch{1..4} (4 alike) : Switch  Criteria=u2 ~= 0  Threshold=0.5  SaturateOnIntegerOverflow=on
  w0 : Constant
  delta : Outport
  w : Outport  Port=2
  wires:
  [Trip] -> Switch3/2, Switch2/2
  Constant1/1 -> Switch3/1, Switch2/1
  Switch3/1 -> Scope4/1, Sum3/1, w/1
  Int2/1 -> Switch3/3
  Switch2/1 -> Int2/1
  Gain1/1 -> Switch2/3
  Trip/1 -> [Trip]
  [Trip] -> Switch1/2, Switch4/2
  Constant2/1 -> Switch4/1, Switch1/1
  Switch4/1 -> delta/1, Scope2/1, Gain5/1
  Int1/1 -> Switch4/3
  Switch1/1 -> Int1/1
  Gain/1 -> Switch1/3
  Gain5/1 -> Scope8/1
  w0/1 -> Sum3/2
  Sum3/1 -> Gain2/1, Gain/1
  Pm/1 -> Sum2/2
  Gain2/1 -> Sum2/1
  Sum2/1 -> Gain1/1
  Pe/1 -> Sum2/3
  dPm/1 -> Sum2/4

== system M4B11/Generator3/Output ==
  Igxy1in : Inport
  GBxyin : Inport  Port=2
  deltain : Inport  Port=3
  Pein : Inport  Port=4
  fin : Inport  Port=5
  Vg : Inport  Port=6
  Bus Creator : BusCreator  Inputs=6
  m : Outport
  Igxy1 : Outport  Port=2
  GBxy : Outport  Port=3
  wires:
  Bus Creator/1 -> m/1
  Igxy1in/1 -> Igxy1/1, Bus Creator/1  "Igxy1"
  GBxyin/1 -> GBxy/1, Bus Creator/2  "GBxy"
  deltain/1 -> Bus Creator/3  "delta"
  Pein/1 -> Bus Creator/4  "Pe"
  fin/1 -> Bus Creator/5  "f"
  Vg/1 -> Bus Creator/6  "Vg"

== system M4B11/Generator3/PSS1 ==
  w : Inport
  Trip : Inport  Port=2
  CT : Constant  Value=0
  Constant : Constant  Value=0
  Gain : Gain  Gain=Kpss  SaturateOnIntegerOverflow=on  OutDataTypeStr=Inherit: Same as input  ParamDataTypeStr=Inherit: Same as input
  Saturation : Saturate  UpperLimit=Upmax  LowerLimit=Upmin
  Sum3 : Sum  Inputs=|+-  SaturateOnIntegerOverflow=on
  Switch : Switch  Threshold=0.5  SaturateOnIntegerOverflow=on
  Switch1 : Switch  Threshold=0.5  SaturateOnIntegerOverflow=on
  Transfer Fcn : TransferFcn  Numerator=[Tw_P 0]  Denominator=[Tw_P 1]
  Transfer Fcn1 : TransferFcn  Numerator=[T1_P 1]  Denominator=[T2_P 1]
  Transfer Fcn2 : TransferFcn  Numerator=[T3_P 1]  Denominator=[T4_P 1]
  w0 : Constant
  w1 : Constant  Value=S_PSS
  Upss : Outport
  wires:
  Constant/1 -> Switch1/1
  Trip/1 -> Switch1/2
  Switch1/1 -> Upss/1
  Switch/1 -> Switch1/3
  Transfer Fcn/1 -> Transfer Fcn1/1
  Gain/1 -> Transfer Fcn/1
  w1/1 -> Switch/2
  CT/1 -> Switch/3
  Saturation/1 -> Switch/1
  Sum3/1 -> Gain/1
  Transfer Fcn2/1 -> Saturation/1
  Transfer Fcn1/1 -> Transfer Fcn2/1
  w/1 -> Sum3/1
  w0/1 -> Sum3/2

== system M4B11/Generator4/Excitation System ==
  note: Ef
  Upss : Inport
  Trip : Inport  Port=2
  Vg : Inport  Port=3
  Constant : Constant  Value=0
  KA : Gain  Gain=Ka  SaturateOnIntegerOverflow=on  OutDataTypeStr=Inherit: Same as input  ParamDataTypeStr=Inherit: Same as input
  Saturation : Saturate  UpperLimit=Efmax  LowerLimit=Efmin
  Scope : Scope  NumInputPorts=2
  Sum4 : Sum  Inputs=+-+  SaturateOnIntegerOverflow=on
  Switch : Switch  Criteria=u2 ~= 0  Threshold=0.5  SaturateOnIntegerOverflow=on
  Vref : Constant  Value=Vref
  Ef : Outport
  wires:
  Trip/1 -> Switch/2
  Constant/1 -> Switch/1
  Switch/1 -> Ef/1
  Saturation/1 -> Switch/3
  Sum4/1 -> KA/1
  KA/1 -> Saturation/1
  Vg/1 -> Sum4/2, Scope/2
  Upss/1 -> Sum4/3
  Vref/1 -> Scope/1, Sum4/1

== system M4B11/Generator4/Governor ==
  w : Inport
  Trip : Inport  Port=2
  CT : Constant  Value=0
  Constant : Constant  Value=0
  Gain1 : Gain  Gain=1/R  SaturateOnIntegerOverflow=on  OutDataTypeStr=Inherit: Same as input  ParamDataTypeStr=Inherit: Same as input
  Saturation : Saturate  UpperLimit=dPmax  LowerLimit=dPmin
  Sum3 : Sum  Inputs=|+-  SaturateOnIntegerOverflow=on
  Switch : Switch  Threshold=0.5  SaturateOnIntegerOverflow=on
  Switch1 : Switch  Criteria=u2 ~= 0  Threshold=0.5  SaturateOnIntegerOverflow=on
  Transfer Fcn1 : TransferFcn  Denominator=[Ts_G 1]
  Transfer Fcn2 : TransferFcn  Numerator=[T3_G 1]  Denominator=[Tc_G 1]
  Transfer Fcn3 : TransferFcn  Numerator=[T4_G 1]  Denominator=[T5_G 1]
  w1 : Constant  Value=S_Gov
  wref : Constant
  dPm : Outport
  wires:
  Constant/1 -> Switch1/1
  Switch/1 -> Switch1/3
  Trip/1 -> Switch1/2
  Switch1/1 -> dPm/1
  CT/1 -> Switch/3
  w1/1 -> Switch/2
  wref/1 -> Sum3/1
  w/1 -> Sum3/2
  Saturation/1 -> Switch/1
  Sum3/1 -> Gain1/1
  Gain1/1 -> Transfer Fcn1/1
  Transfer Fcn1/1 -> Transfer Fcn2/1
  Transfer Fcn2/1 -> Transfer Fcn3/1
  Transfer Fcn3/1 -> Saturation/1

== system M4B11/Generator4/Machine Equations  ==
  note: Idg
  note: Iqg
  delta : Inport
  Vgxy : Inport  Port=2
  Ef : Inport  Port=3
  Trip : Inport  Port=4
  Demux : Demux  Outputs=2
  Demux1 : Demux  Outputs=2
  Fcn1 : Fcn  Expr=u(1)*u(3)+u(2)*u(4)
  Fcn2 : Fcn  Expr=(u(3)-u(2))/Xd11
  Fcn3 : Fcn  Expr=(u(1)-u(4))/Xq11
  Fcn4 : Fcn  Expr=u(2)*u(3)-u(1)*u(4)
  Fcn6 : Fcn  Expr=sqrt(u(1)^2+u(2)^2)
  Interface : Subsystem
  Mux1 : Mux  Inputs=2
  Mux2 : Mux  Inputs=2
  Mux3 : Mux  Inputs=2
  Qe : Scope
  Scope{,1..3} (4 alike) : Scope
  Transient Equations : Subsystem
  Pe : Outport
  Igxy1 : Outport  Port=2
  GBxy : Outport  Port=3
  Vg : Outport  Port=4
  wires:
  Fcn3/1 -> Mux3/2
  Fcn2/1 -> Mux3/1
  Mux3/1 -> Demux1/1, Mux2/2, Transient Equations/1(Idqg)
  Interface/1(Vdqg) -> Demux/1, Mux2/1, Fcn6/1, Mux1/1
  Mux1/1 -> Fcn2/1, Fcn3/1
  Mux2/1 -> Fcn1/1, Fcn4/1
  Ef/1 -> Transient Equations/2(Ef)
  Fcn1/1 -> Pe/1
  Fcn6/1 -> Vg/1
  Fcn4/1 -> Qe/1
  delta/1 -> Interface/1(delta)
  Vgxy/1 -> Interface/2(Vgxy)
  Interface/2(Igxy1) -> Igxy1/1
  Interface/3(GBxy) -> GBxy/1
  Transient Equations/1(Eqd'') -> Mux1/2, Interface/3(Eqd'')
  Demux/1 -> Scope1/1
  Demux1/1 -> Scope/1
  Demux/2 -> Scope2/1
  Demux1/2 -> Scope3/1
  Trip/1 -> [Trip]
  [Trip] -> Transient Equations/3(Trip)

== system M4B11/Generator4/Mechanical DE ==
  Pe : Inport
  dPm : Inport  Port=2
  Trip : Inport  Port=3
  Constant1 : Constant  Value=0
  Constant2 : Constant  Value=0
  Gain : Gain  Gain=wB  SaturateOnIntegerOverflow=on  OutDataTypeStr=Inherit: Same as input  ParamDataTypeStr=Inherit: Same as input
  Gain1 : Gain  Gain=1/H  SaturateOnIntegerOverflow=on  OutDataTypeStr=Inherit: Same as input  ParamDataTypeStr=Inherit: Same as input
  Gain2 : Gain  Gain=D  SaturateOnIntegerOverflow=on  OutDataTypeStr=Inherit: Same as input  ParamDataTypeStr=Inherit: Same as input
  Gain5 : Gain  Gain=180/pi  SaturateOnIntegerOverflow=on  OutDataTypeStr=Inherit: Same as input  ParamDataTypeStr=Inherit: Same as input
  Int1 : Integrator  InitialCondition=delta0
  Int2 : Integrator  InitialCondition=w0
  Pm : Constant  Value=Pm0
  Scope2 : Scope
  Scope4 : Scope
  Scope8 : Scope
  Sum2 : Sum  Inputs=-+-+  SaturateOnIntegerOverflow=on
  Sum3 : Sum  Inputs=|+-  SaturateOnIntegerOverflow=on
  Switch{1..4} (4 alike) : Switch  Criteria=u2 ~= 0  Threshold=0.5  SaturateOnIntegerOverflow=on
  w0 : Constant
  delta : Outport
  w : Outport  Port=2
  wires:
  [Trip] -> Switch3/2, Switch2/2
  Constant1/1 -> Switch3/1, Switch2/1
  Switch3/1 -> Scope4/1, Sum3/1, w/1
  Int2/1 -> Switch3/3
  Switch2/1 -> Int2/1
  Gain1/1 -> Switch2/3
  Trip/1 -> [Trip]
  [Trip] -> Switch1/2, Switch4/2
  Constant2/1 -> Switch4/1, Switch1/1
  Switch4/1 -> delta/1, Scope2/1, Gain5/1
  Int1/1 -> Switch4/3
  Switch1/1 -> Int1/1
  Gain/1 -> Switch1/3
  Gain5/1 -> Scope8/1
  w0/1 -> Sum3/2
  Sum3/1 -> Gain2/1, Gain/1
  Pm/1 -> Sum2/2
  Gain2/1 -> Sum2/1
  Sum2/1 -> Gain1/1
  Pe/1 -> Sum2/3
  dPm/1 -> Sum2/4

== system M4B11/Generator4/Output ==
  Igxy1in : Inport
  GBxyin : Inport  Port=2
  deltain : Inport  Port=3
  Pein : Inport  Port=4
  fin : Inport  Port=5
  Vg : Inport  Port=6
  Bus Creator : BusCreator  Inputs=6
  m : Outport
  Igxy1 : Outport  Port=2
  GBxy : Outport  Port=3
  wires:
  Bus Creator/1 -> m/1
  Igxy1in/1 -> Igxy1/1, Bus Creator/1  "Igxy1"
  GBxyin/1 -> GBxy/1, Bus Creator/2  "GBxy"
  deltain/1 -> Bus Creator/3  "delta"
  Pein/1 -> Bus Creator/4  "Pe"
  fin/1 -> Bus Creator/5  "f"
  Vg/1 -> Bus Creator/6  "Vg"

== system M4B11/Generator4/PSS1 ==
  w : Inport
  Trip : Inport  Port=2
  CT : Constant  Value=0
  Constant : Constant  Value=0
  Gain : Gain  Gain=Kpss  SaturateOnIntegerOverflow=on  OutDataTypeStr=Inherit: Same as input  ParamDataTypeStr=Inherit: Same as input
  Saturation : Saturate  UpperLimit=Upmax  LowerLimit=Upmin
  Sum3 : Sum  Inputs=|+-  SaturateOnIntegerOverflow=on
  Switch : Switch  Threshold=0.5  SaturateOnIntegerOverflow=on
  Switch1 : Switch  Threshold=0.5  SaturateOnIntegerOverflow=on
  Transfer Fcn : TransferFcn  Numerator=[Tw_P 0]  Denominator=[Tw_P 1]
  Transfer Fcn1 : TransferFcn  Numerator=[T1_P 1]  Denominator=[T2_P 1]
  Transfer Fcn2 : TransferFcn  Numerator=[T3_P 1]  Denominator=[T4_P 1]
  w0 : Constant
  w1 : Constant  Value=S_PSS
  Upss : Outport
  wires:
  Constant/1 -> Switch1/1
  Trip/1 -> Switch1/2
  Switch1/1 -> Upss/1
  Switch/1 -> Switch1/3
  Transfer Fcn/1 -> Transfer Fcn1/1
  Gain/1 -> Transfer Fcn/1
  w1/1 -> Switch/2
  CT/1 -> Switch/3
  Saturation/1 -> Switch/1
  Sum3/1 -> Gain/1
  Transfer Fcn2/1 -> Saturation/1
  Transfer Fcn1/1 -> Transfer Fcn2/1
  w/1 -> Sum3/1
  w0/1 -> Sum3/2

== system M4B11/Generator1/Machine Equations /Interface ==
  delta : Inport
  Vgxy : Inport  Port=2
  Eqd'' : Inport  Port=3
  Bx : Fcn  Expr=1/Xq11+(1/Xd11-1/Xq11)*sin(u(1))*sin(u(1))
  By : Fcn  Expr=-1/Xq11-(1/Xd11-1/Xq11)*cos(u(1))*cos(u(1))
  Gx : Fcn  Expr=(1/Xd11-1/Xq11)*sin(u(1))*cos(u(1))
  Gy : Fcn  Expr=(1/Xq11-1/Xd11)*sin(u(1))*cos(u(1))
  Igx1 : Fcn  Expr=sin(u(1))*u(2)/Xd11-cos(u(1))*u(3)/Xq11
  Igy1 : Fcn  Expr=-cos(u(1))*u(2)/Xd11-sin(u(1))*u(3)/Xq11
  Mux{1..3,5} (4 alike) : Mux  Inputs=2
  Mux4 : Mux
  Scope1 : Scope
  Vdg : Fcn  Expr=u(1)*sin(u(3))-u(2)*cos(u(3))
  Vqg : Fcn  Expr=u(1)*cos(u(3))+u(2)*sin(u(3))
  Vdqg : Outport
  Igxy1 : Outport  Port=2
  GBxy : Outport  Port=3
  wires:
  Vgxy/1 -> Mux1/1
  delta/1 -> By/1, Bx/1, Gy/1, Gx/1, Mux1/2, Mux5/1
  Eqd''/1 -> Mux5/2
  Vdg/1 -> Scope1/1, Mux2/1
  Vqg/1 -> Mux2/2
  Mux2/1 -> Vdqg/1
  Igx1/1 -> Mux3/1
  Igy1/1 -> Mux3/2
  Mux3/1 -> Igxy1/1
  Gx/1 -> Mux4/1
  Gy/1 -> Mux4/2
  Bx/1 -> Mux4/3
  By/1 -> Mux4/4
  Mux4/1 -> GBxy/1
  Mux1/1 -> Vdg/1, Vqg/1
  Mux5/1 -> Igx1/1, Igy1/1

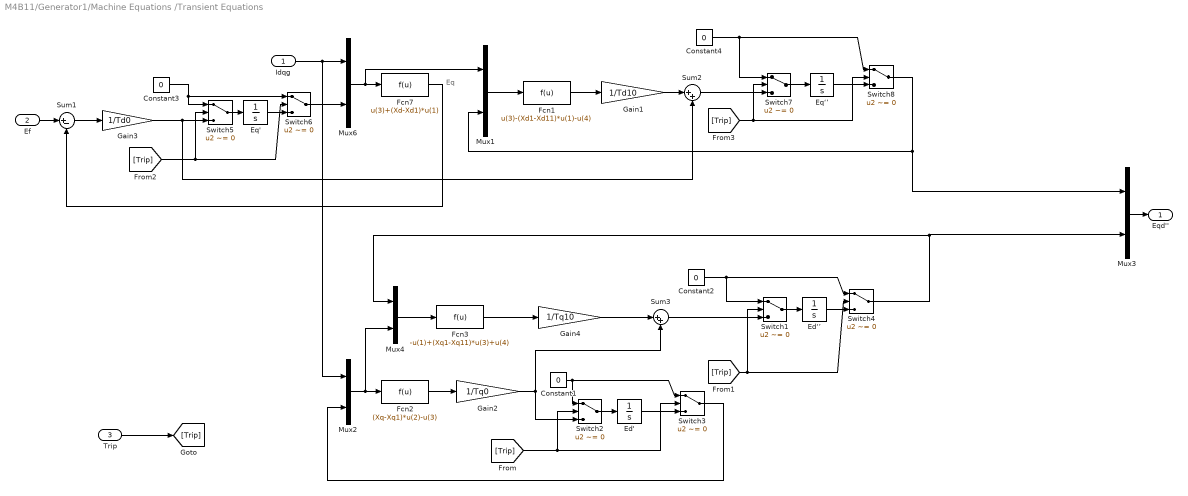
== system M4B11/Generator1/Machine Equations /Transient Equations ==
  note: Eq
  Idqg : Inport
  Ef : Inport  Port=2
  Trip : Inport  Port=3
  Constant{1..4} (4 alike) : Constant  Value=0
  Ed' : Integrator  InitialCondition=Ed10
  Ed‘’ : Integrator  InitialCondition=Ed110
  Eq' : Integrator  InitialCondition=Eq10
  Eq‘’ : Integrator  InitialCondition=Eq110
  Fcn1 : Fcn  Expr=u(3)-(Xd1-Xd11)*u(1)-u(4)
  Fcn2 : Fcn  Expr=(Xq-Xq1)*u(2)-u(3)
  Fcn3 : Fcn  Expr=-u(1)+(Xq1-Xq11)*u(3)+u(4)
  Fcn7 : Fcn  Expr=u(3)+(Xd-Xd1)*u(1)
  Gain1 : Gain  Gain=1/Td10  SaturateOnIntegerOverflow=on  OutDataTypeStr=Inherit: Same as input  ParamDataTypeStr=Inherit: Same as input
  Gain2 : Gain  Gain=1/Tq0  SaturateOnIntegerOverflow=on  OutDataTypeStr=Inherit: Same as input  ParamDataTypeStr=Inherit: Same as input
  Gain3 : Gain  Gain=1/Td0  SaturateOnIntegerOverflow=on  OutDataTypeStr=Inherit: Same as input  ParamDataTypeStr=Inherit: Same as input
  Gain4 : Gain  Gain=1/Tq10  SaturateOnIntegerOverflow=on  OutDataTypeStr=Inherit: Same as input  ParamDataTypeStr=Inherit: Same as input
  Mux{1..4,6} (5 alike) : Mux  Inputs=2
  Sum1 : Sum  Inputs=|+-  SaturateOnIntegerOverflow=on
  Sum2 : Sum  Inputs=|++  SaturateOnIntegerOverflow=on
  Sum3 : Sum  Inputs=|++  SaturateOnIntegerOverflow=on
  Switch{1..8} (8 alike) : Switch  Criteria=u2 ~= 0  Threshold=0.5  SaturateOnIntegerOverflow=on
  Eqd'' : Outport
  wires:
  Gain3/1 -> Sum2/2, Switch5/3
  Sum1/1 -> Gain3/1
  Mux6/1 -> Fcn7/1, Mux1/1
  Fcn7/1 -> Sum1/2
  Idqg/1 -> Mux2/1, Mux6/1
  Ef/1 -> Sum1/1
  Gain1/1 -> Sum2/1
  Fcn1/1 -> Gain1/1
  Mux1/1 -> Fcn1/1
  Mux2/1 -> Fcn2/1, Mux4/2
  Fcn2/1 -> Gain2/1
  Gain2/1 -> Switch2/3, Sum3/2
  Mux3/1 -> Eqd''/1
  Gain4/1 -> Sum3/1
  Fcn3/1 -> Gain4/1
  Mux4/1 -> Fcn3/1
  Constant1/1 -> Switch2/1, Switch3/1
  Switch2/1 -> Ed'/1
  Ed'/1 -> Switch3/3
  Switch3/1 -> Mux2/2
  Trip/1 -> [Trip]
  [Trip] -> Switch3/2, Switch2/2
  Sum3/1 -> Switch1/3
  Switch1/1 -> Ed‘’/1
  Ed‘’/1 -> Switch4/3
  Switch4/1 -> Mux4/1, Mux3/2
  Constant2/1 -> Switch1/1, Switch4/1
  [Trip] -> Switch4/2, Switch1/2
  Switch5/1 -> Eq'/1
  Eq'/1 -> Switch6/3
  Switch6/1 -> Mux6/2
  Constant3/1 -> Switch6/1, Switch5/1
  [Trip] -> Switch6/2, Switch5/2
  Sum2/1 -> Switch7/3
  Switch7/1 -> Eq‘’/1
  Switch8/1 -> Mux1/2, Mux3/1
  Eq‘’/1 -> Switch8/3
  [Trip] -> Switch8/2, Switch7/2
  Constant4/1 -> Switch7/1, Switch8/1

== system M4B11/Generator2/Machine Equations /Interface ==
  delta : Inport
  Vgxy : Inport  Port=2
  Eqd'' : Inport  Port=3
  Bx : Fcn  Expr=1/Xq11+(1/Xd11-1/Xq11)*sin(u(1))*sin(u(1))
  By : Fcn  Expr=-1/Xq11-(1/Xd11-1/Xq11)*cos(u(1))*cos(u(1))
  Gx : Fcn  Expr=(1/Xd11-1/Xq11)*sin(u(1))*cos(u(1))
  Gy : Fcn  Expr=(1/Xq11-1/Xd11)*sin(u(1))*cos(u(1))
  Igx1 : Fcn  Expr=sin(u(1))*u(2)/Xd11-cos(u(1))*u(3)/Xq11
  Igy1 : Fcn  Expr=-cos(u(1))*u(2)/Xd11-sin(u(1))*u(3)/Xq11
  Mux{1..3,5} (4 alike) : Mux  Inputs=2
  Mux4 : Mux
  Scope1 : Scope
  Vdg : Fcn  Expr=u(1)*sin(u(3))-u(2)*cos(u(3))
  Vqg : Fcn  Expr=u(1)*cos(u(3))+u(2)*sin(u(3))
  Vdqg : Outport
  Igxy1 : Outport  Port=2
  GBxy : Outport  Port=3
  wires:
  Vgxy/1 -> Mux1/1
  delta/1 -> By/1, Bx/1, Gy/1, Gx/1, Mux1/2, Mux5/1
  Eqd''/1 -> Mux5/2
  Vdg/1 -> Scope1/1, Mux2/1
  Vqg/1 -> Mux2/2
  Mux2/1 -> Vdqg/1
  Igx1/1 -> Mux3/1
  Igy1/1 -> Mux3/2
  Mux3/1 -> Igxy1/1
  Gx/1 -> Mux4/1
  Gy/1 -> Mux4/2
  Bx/1 -> Mux4/3
  By/1 -> Mux4/4
  Mux4/1 -> GBxy/1
  Mux1/1 -> Vdg/1, Vqg/1
  Mux5/1 -> Igx1/1, Igy1/1

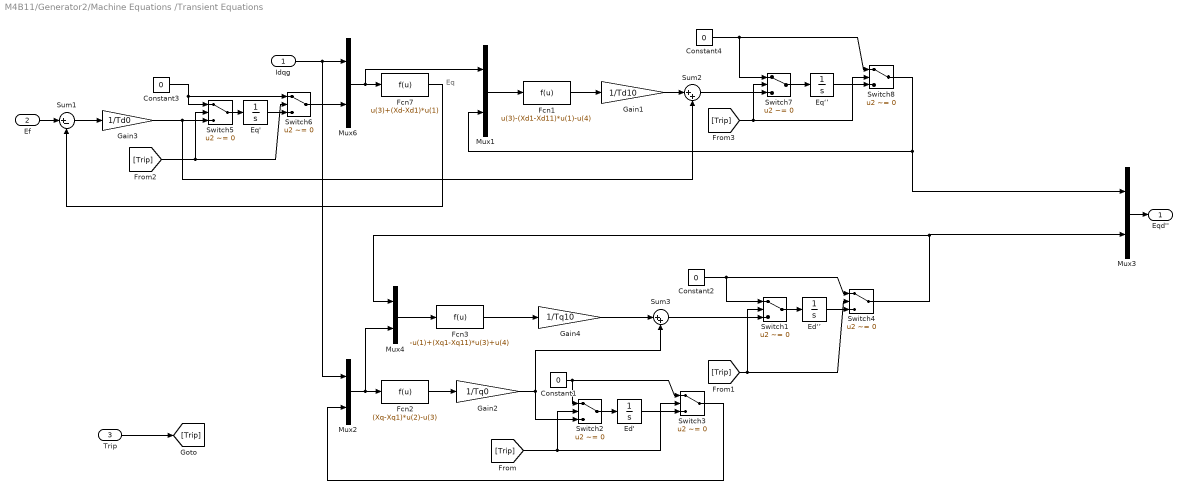
== system M4B11/Generator2/Machine Equations /Transient Equations ==
  note: Eq
  Idqg : Inport
  Ef : Inport  Port=2
  Trip : Inport  Port=3
  Constant{1..4} (4 alike) : Constant  Value=0
  Ed' : Integrator  InitialCondition=Ed10
  Ed‘’ : Integrator  InitialCondition=Ed110
  Eq' : Integrator  InitialCondition=Eq10
  Eq‘’ : Integrator  InitialCondition=Eq110
  Fcn1 : Fcn  Expr=u(3)-(Xd1-Xd11)*u(1)-u(4)
  Fcn2 : Fcn  Expr=(Xq-Xq1)*u(2)-u(3)
  Fcn3 : Fcn  Expr=-u(1)+(Xq1-Xq11)*u(3)+u(4)
  Fcn7 : Fcn  Expr=u(3)+(Xd-Xd1)*u(1)
  Gain1 : Gain  Gain=1/Td10  SaturateOnIntegerOverflow=on  OutDataTypeStr=Inherit: Same as input  ParamDataTypeStr=Inherit: Same as input
  Gain2 : Gain  Gain=1/Tq0  SaturateOnIntegerOverflow=on  OutDataTypeStr=Inherit: Same as input  ParamDataTypeStr=Inherit: Same as input
  Gain3 : Gain  Gain=1/Td0  SaturateOnIntegerOverflow=on  OutDataTypeStr=Inherit: Same as input  ParamDataTypeStr=Inherit: Same as input
  Gain4 : Gain  Gain=1/Tq10  SaturateOnIntegerOverflow=on  OutDataTypeStr=Inherit: Same as input  ParamDataTypeStr=Inherit: Same as input
  Mux{1..4,6} (5 alike) : Mux  Inputs=2
  Sum1 : Sum  Inputs=|+-  SaturateOnIntegerOverflow=on
  Sum2 : Sum  Inputs=|++  SaturateOnIntegerOverflow=on
  Sum3 : Sum  Inputs=|++  SaturateOnIntegerOverflow=on
  Switch{1..8} (8 alike) : Switch  Criteria=u2 ~= 0  Threshold=0.5  SaturateOnIntegerOverflow=on
  Eqd'' : Outport
  wires:
  Gain3/1 -> Sum2/2, Switch5/3
  Sum1/1 -> Gain3/1
  Mux6/1 -> Fcn7/1, Mux1/1
  Fcn7/1 -> Sum1/2
  Idqg/1 -> Mux2/1, Mux6/1
  Ef/1 -> Sum1/1
  Gain1/1 -> Sum2/1
  Fcn1/1 -> Gain1/1
  Mux1/1 -> Fcn1/1
  Mux2/1 -> Fcn2/1, Mux4/2
  Fcn2/1 -> Gain2/1
  Gain2/1 -> Switch2/3, Sum3/2
  Mux3/1 -> Eqd''/1
  Gain4/1 -> Sum3/1
  Fcn3/1 -> Gain4/1
  Mux4/1 -> Fcn3/1
  Constant1/1 -> Switch2/1, Switch3/1
  Switch2/1 -> Ed'/1
  Ed'/1 -> Switch3/3
  Switch3/1 -> Mux2/2
  Trip/1 -> [Trip]
  [Trip] -> Switch3/2, Switch2/2
  Sum3/1 -> Switch1/3
  Switch1/1 -> Ed‘’/1
  Ed‘’/1 -> Switch4/3
  Switch4/1 -> Mux4/1, Mux3/2
  Constant2/1 -> Switch1/1, Switch4/1
  [Trip] -> Switch4/2, Switch1/2
  Switch5/1 -> Eq'/1
  Eq'/1 -> Switch6/3
  Switch6/1 -> Mux6/2
  Constant3/1 -> Switch6/1, Switch5/1
  [Trip] -> Switch6/2, Switch5/2
  Sum2/1 -> Switch7/3
  Switch7/1 -> Eq‘’/1
  Switch8/1 -> Mux1/2, Mux3/1
  Eq‘’/1 -> Switch8/3
  [Trip] -> Switch8/2, Switch7/2
  Constant4/1 -> Switch7/1, Switch8/1

== system M4B11/Generator3/Machine Equations /Interface ==
  delta : Inport
  Vgxy : Inport  Port=2
  Eqd'' : Inport  Port=3
  Bx : Fcn  Expr=1/Xq11+(1/Xd11-1/Xq11)*sin(u(1))*sin(u(1))
  By : Fcn  Expr=-1/Xq11-(1/Xd11-1/Xq11)*cos(u(1))*cos(u(1))
  Gx : Fcn  Expr=(1/Xd11-1/Xq11)*sin(u(1))*cos(u(1))
  Gy : Fcn  Expr=(1/Xq11-1/Xd11)*sin(u(1))*cos(u(1))
  Igx1 : Fcn  Expr=sin(u(1))*u(2)/Xd11-cos(u(1))*u(3)/Xq11
  Igy1 : Fcn  Expr=-cos(u(1))*u(2)/Xd11-sin(u(1))*u(3)/Xq11
  Mux{1..3,5} (4 alike) : Mux  Inputs=2
  Mux4 : Mux
  Scope1 : Scope
  Vdg : Fcn  Expr=u(1)*sin(u(3))-u(2)*cos(u(3))
  Vqg : Fcn  Expr=u(1)*cos(u(3))+u(2)*sin(u(3))
  Vdqg : Outport
  Igxy1 : Outport  Port=2
  GBxy : Outport  Port=3
  wires:
  Vgxy/1 -> Mux1/1
  delta/1 -> By/1, Bx/1, Gy/1, Gx/1, Mux1/2, Mux5/1
  Eqd''/1 -> Mux5/2
  Vdg/1 -> Scope1/1, Mux2/1
  Vqg/1 -> Mux2/2
  Mux2/1 -> Vdqg/1
  Igx1/1 -> Mux3/1
  Igy1/1 -> Mux3/2
  Mux3/1 -> Igxy1/1
  Gx/1 -> Mux4/1
  Gy/1 -> Mux4/2
  Bx/1 -> Mux4/3
  By/1 -> Mux4/4
  Mux4/1 -> GBxy/1
  Mux1/1 -> Vdg/1, Vqg/1
  Mux5/1 -> Igx1/1, Igy1/1
